simulink model "Lazo_Abierto"  (R2024b)
settings: Solver=ode15s  StartTime=0.0  StopTime=10.0  MaxStep=1e-3  RelTol=1e-3
settings Model: Creator=leslie  LastModifiedBy=leslie
settings DataIOCC: ReturnWorkspaceOutputs=off  TimeSaveName=t  OutputSaveName=y
settings DebuggingCC: AlgebraicLoopMsg=none  ArtificialAlgebraicLoopMsg=none  MaxConsecutiveZCsMsg=none  OperatingPointInterfaceChecksumMismatchMsg=none

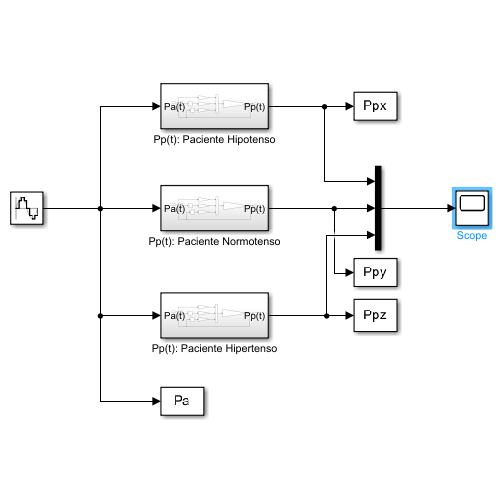
[thumbnail: Simulink's stored preview of the top-level diagram]
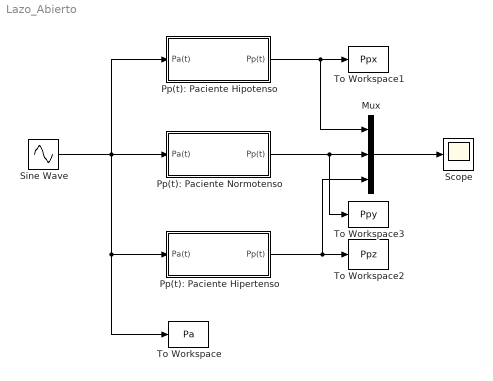
== system Lazo_Abierto ==
  Mux : Mux  Inputs=3
  Pp(t): Paciente Hipertenso : Subsystem
  Pp(t): Paciente Hipotenso : Subsystem
  Pp(t): Paciente Normotenso : Subsystem
  Scope : Scope
  Sine Wave : Sin  Bias=0.8  Frequency=(2*pi)*(95/60)  SampleTime=0.001
  To Workspace : ToWorkspace  VariableName=Pa  SaveFormat=Timeseries  SampleTime=-1
  To Workspace1 : ToWorkspace  VariableName=Ppx  SaveFormat=Timeseries  SampleTime=-1
  To Workspace2 : ToWorkspace  VariableName=Ppz  SaveFormat=Timeseries  SampleTime=-1
  To Workspace3 : ToWorkspace  VariableName=Ppy  SaveFormat=Timeseries  SampleTime=-1
  wires:
  Mux/1 -> Scope/1
  Sine Wave/1 -> Pp(t): Paciente Hipotenso/1(Pa(t)), Pp(t): Paciente Normotenso/1(Pa(t)), To Workspace/1, Pp(t): Paciente Hipertenso/1(Pa(t))
  Pp(t): Paciente Hipotenso/1(Pp(t)) -> To Workspace1/1, Mux/1
  Pp(t): Paciente Normotenso/1(Pp(t)) -> To Workspace3/1, Mux/2
  Pp(t): Paciente Hipertenso/1(Pp(t)) -> Mux/3, To Workspace2/1

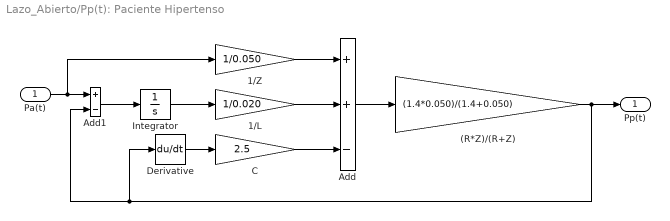
== system Lazo_Abierto/Pp(t): Paciente Hipertenso ==
  Pa(t) : Inport
  (R*Z)/(R+Z) : Gain  Gain=(1.4*0.050)/(1.4+0.050)
  1/L : Gain  Gain=1/0.020
  1/Z : Gain  Gain=1/0.050
  Add : Sum  Inputs=++-
  Add1 : Sum  Inputs=+-
  C : Gain  Gain=2.5
  Derivative : Derivative
  Integrator : Integrator
  Pp(t) : Outport
  wires:
  Add/1 -> (R*Z)/(R+Z)/1
  Derivative/1 -> C/1
  1/Z/1 -> Add/1
  C/1 -> Add/3
  1/L/1 -> Add/2
  Integrator/1 -> 1/L/1
  Pa(t)/1 -> 1/Z/1, Add1/1
  (R*Z)/(R+Z)/1 -> Pp(t)/1, Derivative/1, Add1/2
  Add1/1 -> Integrator/1

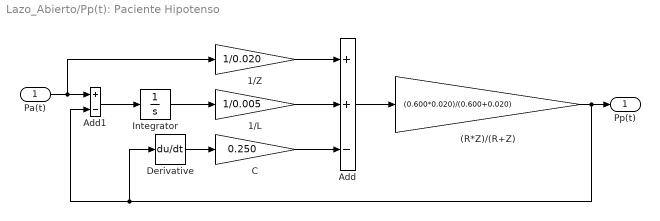
== system Lazo_Abierto/Pp(t): Paciente Hipotenso ==
  Pa(t) : Inport
  (R*Z)/(R+Z) : Gain  Gain=(0.600*0.020)/(0.600+0.020)
  1/L : Gain  Gain=1/0.005
  1/Z : Gain  Gain=1/0.020
  Add : Sum  Inputs=++-
  Add1 : Sum  Inputs=+-
  C : Gain  Gain=0.250
  Derivative : Derivative
  Integrator : Integrator
  Pp(t) : Outport
  wires:
  1/Z/1 -> Add/1
  1/L/1 -> Add/2
  C/1 -> Add/3
  Derivative/1 -> C/1
  Integrator/1 -> 1/L/1
  Add1/1 -> Integrator/1
  Pa(t)/1 -> 1/Z/1, Add1/1
  Add/1 -> (R*Z)/(R+Z)/1
  (R*Z)/(R+Z)/1 -> Derivative/1, Add1/2, Pp(t)/1

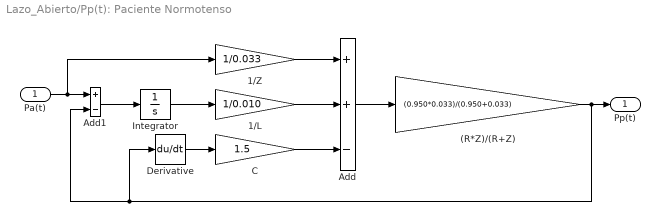
== system Lazo_Abierto/Pp(t): Paciente Normotenso ==
  Pa(t) : Inport
  (R*Z)/(R+Z) : Gain  Gain=(0.950*0.033)/(0.950+0.033)
  1/L : Gain  Gain=1/0.010
  1/Z : Gain  Gain=1/0.033
  Add : Sum  Inputs=++-
  Add1 : Sum  Inputs=+-
  C : Gain  Gain=1.5
  Derivative : Derivative
  Integrator : Integrator
  Pp(t) : Outport
  wires:
  Add/1 -> (R*Z)/(R+Z)/1
  Derivative/1 -> C/1
  1/Z/1 -> Add/1
  C/1 -> Add/3
  1/L/1 -> Add/2
  Integrator/1 -> 1/L/1
  Pa(t)/1 -> 1/Z/1, Add1/1
  (R*Z)/(R+Z)/1 -> Pp(t)/1, Derivative/1, Add1/2
  Add1/1 -> Integrator/1
